simulink model "quadDyanamics"  (Simulink 2.20)
settings: Solver=ode45  StartTime=0.0  StopTime=10  RelTol=1e-3  AbsTol=1e-6
CloseFcn:
  | ;slview('closediagram',bdroot);;slview('closediagram',bdroot);;slview('closediagram',bdroot);
settings Model: ConsistencyChecking=off  RTWPlaceOutputsASAP=off

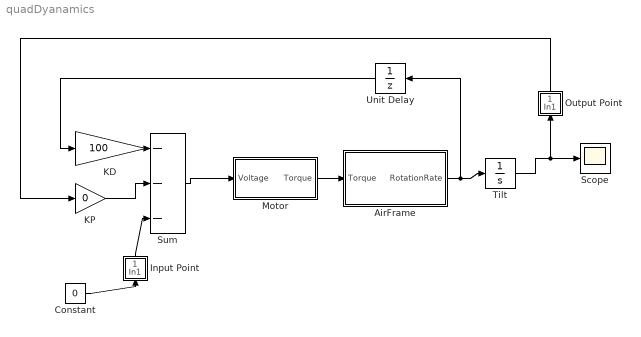
== system quadDyanamics ==
  AirFrame : Subsystem
  Constant : Constant  Value=0
  Input Point : Subsystem  Orientation=up
      settings: CopyFcn=connectline('copy');  DeleteFcn=connectline('delete');  OpenFcn=connectline('open');
      mask Type: InputPoint
      mask Display: plot(33,-30,66,100,[31,38],[70,70],[34.5,34.5],[56,86],[50,50],[50,100],[50,55],[50,80],[50,45],[50,80],[50,53,55,55,55,53,50,47,44,44,44,47,50],[50,49,40,30,21,10,10,10,21,30,40,50,50],[33 44],[31 31],[56 66],[31 31])
  KD : Gain  Gain=100
  KP : Gain  Gain=0
  Motor : Subsystem
  Output Point : Subsystem  Orientation=up
      settings: CopyFcn=connectline('copy');  DeleteFcn=connectline('delete');  OpenFcn=connectline('open');
      mask Type: OutputPoint
      mask Display: plot(33,-30,66,100,[49.5,49.5],[50,100],[50,55],[100,80],[50,45],[100,80],[46,48,51,53,53,50,48,46,46],[40,50,50,40,30,20,21,30,40],[33 44],[33 33],[53 66],[33 33])
  Scope : Scope
      settings: TickLabels=on  TimeRange=auto  YMin=-5  YMax=5  SaveToWorkspace=off  SaveName=ScopeData
  Sum : Sum  Inputs=---
  Tilt : Integrator  ExternalReset=none  InitialConditionSource=internal  InitialCondition=0  LimitOutput=off  UpperSaturationLimit=inf  LowerSaturationLimit=-inf  ShowSaturationPort=off  ShowStatePort=off  AbsoluteTolerance=auto
  Unit Delay : UnitDelay  Orientation=left  X0=1  SampleTime=0.04
  wires:
  Motor/1(Torque) -> AirFrame/1(Torque)
  Sum/1 -> Motor/1(Voltage)
  KD/1 -> Sum/1
  KP/1 -> Sum/2
  Tilt/1 -> Scope/1, Output Point/1(In1)
  AirFrame/1(RotationRate) -> Tilt/1, Unit Delay/1
  Unit Delay/1 -> KD/1
  Constant/1 -> Input Point/1(In1)
  Input Point/1(Out1) -> Sum/3
  Output Point/1(Out1) -> KP/1

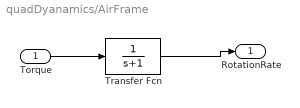
== system quadDyanamics/AirFrame ==
  Torque : Inport  Port=1  PortWidth=-1  SampleTime=-1
  Transfer Fcn : TransferFcn  Numerator=[1]  Denominator=[1 1]
  RotationRate : Outport  Port=1
  wires:
  Torque/1 -> Transfer Fcn/1
  Transfer Fcn/1 -> RotationRate/1

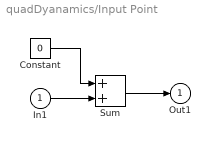
== system quadDyanamics/Input Point ==
  In1 : Inport  Port=1  PortWidth=-1  SampleTime=-1
  Constant : Constant  Value=0
  Sum : Sum  Inputs=++
  Out1 : Outport  Port=1  InitialOutput=0
  wires:
  Constant/1 -> Sum/1
  Sum/1 -> Out1/1
  In1/1 -> Sum/2

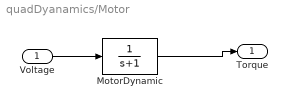
== system quadDyanamics/Motor ==
  Voltage : Inport  Port=1  PortWidth=-1  SampleTime=-1
  MotorDynamic : TransferFcn  Numerator=[1]  Denominator=[1 1]
  Torque : Outport  Port=1
  wires:
  Voltage/1 -> MotorDynamic/1
  MotorDynamic/1 -> Torque/1

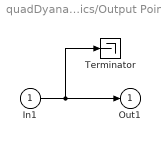
== system quadDyanamics/Output Point ==
  In1 : Inport  Port=1  PortWidth=-1  SampleTime=-1
  Terminator : Terminator
  Out1 : Outport  Port=1  InitialOutput=0
  wires:
  In1/1 -> Terminator/1, Out1/1
